simulink model "APM_sl"  (R2022b)
settings: Solver=VariableStepAuto  StartTime=0.0  StopTime=10.0  RelTol=1e-3
settings Model: Creator=HQ03  LastModifiedBy=HQ03

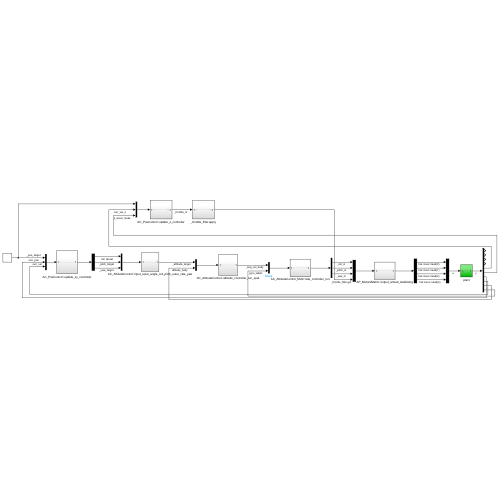
[thumbnail: Simulink's stored preview of the top-level diagram]
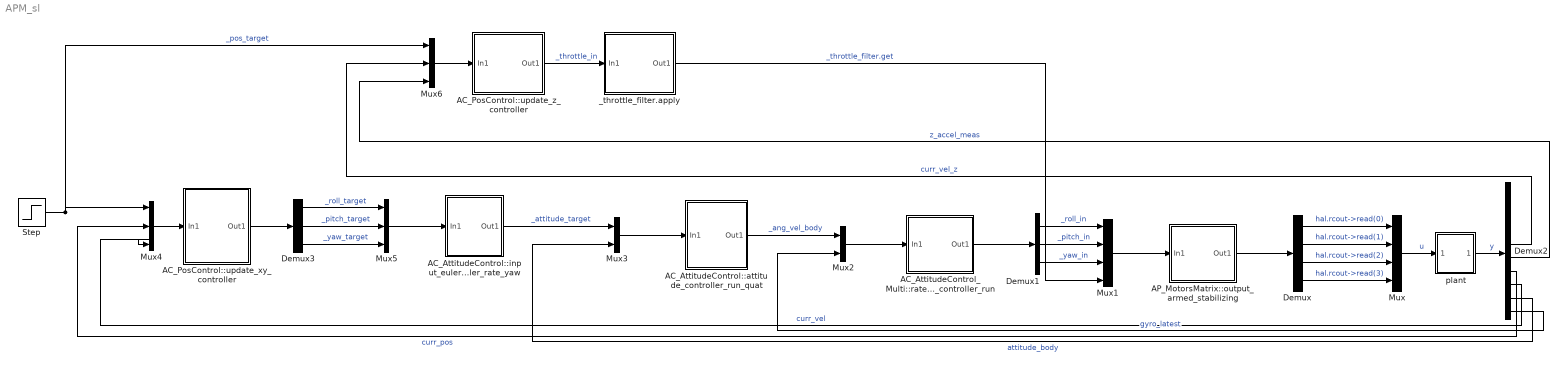
== system APM_sl ==
  AC_AttitudeControl::attitude_controller_run_quat : Subsystem
  AC_AttitudeControl::input_euler_angle_roll_pitch_euler_rate_yaw : Subsystem
  AC_AttitudeControl_Multi::rate_controller_run : Subsystem
  AC_PosControl::update_xy_controller : Subsystem
  AC_PosControl::update_z_controller : Subsystem
  AP_MotorsMatrix::output_armed_stabilizing : Subsystem
  Demux : Demux
  Demux1 : Demux  Outputs=3
  Demux2 : Demux  Outputs=10
  Demux3 : Demux  Outputs=3
  Mux : Mux
  Mux1 : Mux
  Mux2 : Mux  Inputs=2
  Mux3 : Mux  Inputs=2
  Mux4 : Mux  Inputs=3
  Mux5 : Mux  Inputs=3
  Mux6 : Mux  Inputs=3
  Step : Step  SampleTime=0
  _throttle_filter.apply : Subsystem
  plant : Subsystem
  wires:
  Mux/1 -> plant/1(In1)  "u"
  AP_MotorsMatrix::output_armed_stabilizing/1(Out1) -> Demux/1
  Demux/1 -> Mux/1  "hal.rcout->read(0)"
  Demux/2 -> Mux/2  "hal.rcout->read(1)"
  Demux/3 -> Mux/3  "hal.rcout->read(2)"
  Demux/4 -> Mux/4  "hal.rcout->read(3)"
  Mux1/1 -> AP_MotorsMatrix::output_armed_stabilizing/1(In1)
  AC_AttitudeControl_Multi::rate_controller_run/1(Out1) -> Demux1/1
  Demux1/1 -> Mux1/1  "_roll_in"
  Demux1/2 -> Mux1/2  "_pitch_in"
  Demux1/3 -> Mux1/3  "_yaw_in"
  _throttle_filter.apply/1(Out1) -> Mux1/4  "_throttle_filter.get"
  Mux2/1 -> AC_AttitudeControl_Multi::rate_controller_run/1(In1)
  AC_AttitudeControl::attitude_controller_run_quat/1(Out1) -> Mux2/1  "_ang_vel_body"
  plant/1(Out1) -> Demux2/1  "y"
  Mux3/1 -> AC_AttitudeControl::attitude_controller_run_quat/1(In1)
  AC_AttitudeControl::input_euler_angle_roll_pitch_euler_rate_yaw/1(Out1) -> Mux3/1  "_attitude_target"
  Mux4/1 -> AC_PosControl::update_xy_controller/1(In1)
  Step/1 -> Mux4/1, Mux6/1  "_pos_target"
  Demux2/7 -> Mux4/2  "curr_pos"
  AC_PosControl::update_xy_controller/1(Out1) -> Demux3/1
  Demux3/1 -> Mux5/1  "_roll_target"
  Demux3/2 -> Mux5/2  "_pitch_target"
  Demux3/3 -> Mux5/3  "_yaw_target"
  Mux5/1 -> AC_AttitudeControl::input_euler_angle_roll_pitch_euler_rate_yaw/1(In1)
  Demux2/8 -> Mux4/3  "curr_vel"
  Demux2/10 -> Mux2/2  "gyro_latest"
  Demux2/9 -> Mux3/2  "attitude_body"
  Demux2/5 -> Mux6/2  "curr_vel_z"
  Demux2/6 -> Mux6/3  "z_accel_meas"
  Mux6/1 -> AC_PosControl::update_z_controller/1(In1)
  AC_PosControl::update_z_controller/1(Out1) -> _throttle_filter.apply/1(In1)  "_throttle_in"

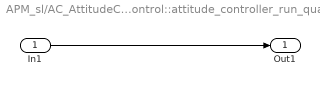
== system APM_sl/AC_AttitudeControl::attitude_controller_run_quat ==
  In1 : Inport
  Out1 : Outport
  wires:
  In1/1 -> Out1/1

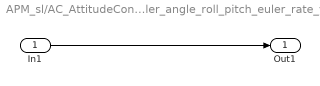
== system APM_sl/AC_AttitudeControl::input_euler_angle_roll_pitch_euler_rate_yaw ==
  In1 : Inport
  Out1 : Outport
  wires:
  In1/1 -> Out1/1

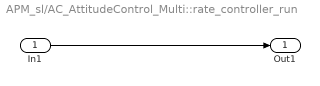
== system APM_sl/AC_AttitudeControl_Multi::rate_controller_run ==
  In1 : Inport
  Out1 : Outport
  wires:
  In1/1 -> Out1/1

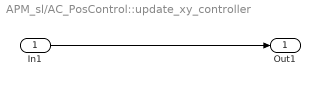
== system APM_sl/AC_PosControl::update_xy_controller ==
  In1 : Inport
  Out1 : Outport
  wires:
  In1/1 -> Out1/1

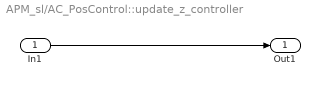
== system APM_sl/AC_PosControl::update_z_controller ==
  In1 : Inport
  Out1 : Outport
  wires:
  In1/1 -> Out1/1

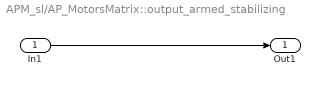
== system APM_sl/AP_MotorsMatrix::output_armed_stabilizing ==
  In1 : Inport
  Out1 : Outport
  wires:
  In1/1 -> Out1/1

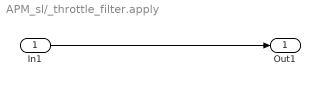
== system APM_sl/_throttle_filter.apply ==
  In1 : Inport
  Out1 : Outport
  wires:
  In1/1 -> Out1/1

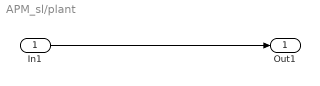
== system APM_sl/plant ==
  In1 : Inport
  Out1 : Outport
  wires:
  In1/1 -> Out1/1
